simulink model "FF_simulink"  (R2018b)
settings: Solver=VariableStepAuto  StartTime=0.0  StopTime=5  RelTol=1e-3
undefined symbols (not defined in the file): alpha, CL, Cm, g, Iyy, m, V
libraries: vrlib x5, simulink_extras x2
settings Model: Creator=ferra  LastModifiedBy=ferra

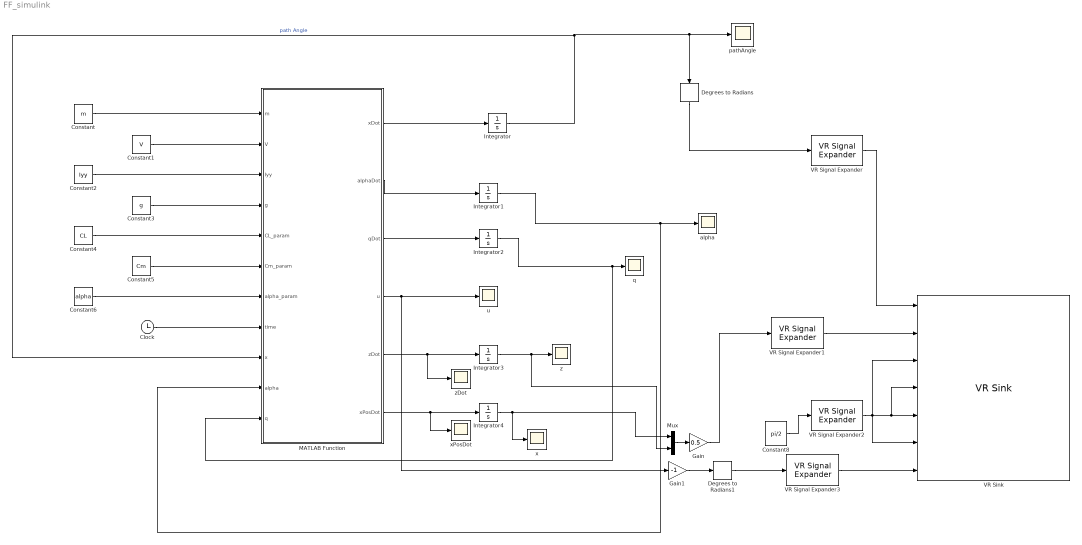
== system FF_simulink ==
  Clock : Clock
  Constant : Constant  Value=m
  Constant1 : Constant  Value=V
  Constant2 : Constant  Value=Iyy
  Constant3 : Constant  Value=g
  Constant4 : Constant  Value=CL
  Constant5 : Constant  Value=Cm
  Constant6 : Constant  Value=alpha
  Constant8 : Constant  Value=pi/2
  Degrees to Radians : simulink_extras/Transformations/Degrees to Radians
  Degrees to Radians1 : simulink_extras/Transformations/Degrees to Radians
  Gain : Gain  Gain=0.5
  Gain1 : Gain  Gain=-1
  Integrator : Integrator
  Integrator1 : Integrator
  Integrator2 : Integrator
  Integrator3 : Integrator  InitialCondition=5
  Integrator4 : Integrator  InitialCondition=-30
  MATLAB Function : MATLAB Function  TreatAsAtomicUnit=on
  Mux : Mux  Inputs=2
  VR Signal Expander : vrlib/VR Signal Expander  outwidth=4  outidx=[4]
      settings: SourceProductName=Simulink 3D Animation  SourceProductBaseCode=VR
  VR Signal Expander1 : vrlib/VR Signal Expander  outwidth=3  outidx=[1 2]
      settings: SourceProductName=Simulink 3D Animation  SourceProductBaseCode=VR
  VR Signal Expander2 : vrlib/VR Signal Expander  outwidth=4  outidx=[4]
      settings: SourceProductName=Simulink 3D Animation  SourceProductBaseCode=VR
  VR Signal Expander3 : vrlib/VR Signal Expander  outwidth=4  outidx=[4]
      settings: SourceProductName=Simulink 3D Animation  SourceProductBaseCode=VR
  VR Sink : vrlib/VR Sink  InstantiateOnLoad=on  SampleTime=0.01  ViewEnable=on  RemoteChange=off  RemoteView=off  FieldsWritten=Airplane.rotation.4.1.1.double#Airplane.translation.3.1.1.double#Rotor_1.rotation.4.1.1.double#Rotor_2.rotation.4.1.1.double#Rotor_3.rotation.4.1.1.double#Rotor_4.rotation.4.1.1.double#Flap_tail.rotation.4.1.1.double  WorldFileName=C:\Users\ferra\Desktop\Projects\Matlab\Thesis\3D-simulation\3D_world.WRL  AutoView=off  VideoDimensions=[]  AllowVariableSize=off
      settings: SourceProductBaseCode=VR
  alpha : Scope
  pathAngle : Scope
  q : Scope
  u : Scope
  x : Scope
  xPosDot : Scope
  "z " : Scope
  zDot : Scope
  wires:
  Constant1/1 -> MATLAB Function/2(V)
  Constant2/1 -> MATLAB Function/3(Iyy)
  Constant3/1 -> MATLAB Function/4(g)
  Constant4/1 -> MATLAB Function/5(CL_param)
  Constant5/1 -> MATLAB Function/6(Cm_param)
  MATLAB Function/1(xDot) -> Integrator/1
  MATLAB Function/2(alphaDot) -> Integrator1/1
  MATLAB Function/3(qDot) -> Integrator2/1
  Integrator/1 -> pathAngle/1, Degrees to Radians/1, MATLAB Function/9(x)  "path Angle"
  Integrator2/1 -> MATLAB Function/11(q), q/1
  Constant6/1 -> MATLAB Function/7(alpha_param)
  MATLAB Function/4(u) -> Gain1/1, u/1
  Clock/1 -> MATLAB Function/8(time)
  Degrees to Radians/1 -> VR Signal Expander/1
  Integrator1/1 -> MATLAB Function/10(alpha), alpha/1
  Constant/1 -> MATLAB Function/1(m)
  MATLAB Function/5(zDot) -> zDot/1, Integrator3/1
  Integrator3/1 -> Mux/2, "z "/1
  MATLAB Function/6(xPosDot) -> xPosDot/1, Integrator4/1
  Integrator4/1 -> Mux/1, x/1
  Mux/1 -> Gain/1
  Gain/1 -> VR Signal Expander1/1
  Constant8/1 -> VR Signal Expander2/1
  VR Signal Expander/1 -> VR Sink/1
  VR Signal Expander1/1 -> VR Sink/2
  VR Signal Expander2/1 -> VR Sink/3, VR Sink/4, VR Sink/5, VR Sink/6
  VR Signal Expander3/1 -> VR Sink/7
  Degrees to Radians1/1 -> VR Signal Expander3/1
  Gain1/1 -> Degrees to Radians1/1

== matlab function FF_simulink/MATLAB Function ==
  data: m input; xDot output; V input; Iyy input; g input; CL_param input; Cm_param input; alpha_param input; time input; alphaDot output; qDot output; x input; alpha input; q input; u output; zDot output; xPosDot output
function [xDot,alphaDot,qDot,u ,zDot , xPosDot ] = FF(m,V,Iyy,g,CL_param,Cm_param,...
                                    alpha_param, time,x,alpha,q)
Cm = mean(Cm_param);
T = 10;


k1 = 2;
k2 = 2;

if(alpha>71)
    alpha = 71;
elseif(alpha<-10)
    alpha = -10;
end



alphaRound = round(alpha*2)/2;

seqIndex = 1:1:length(alpha_param);
index = round(interp1(alpha_param,seqIndex,alphaRound));
CL = CL_param(index);

f = (-g/V) * cos((CL*x)/(m*V));
f1 = (g/V) * cos((CL*x)/(m*V)) - (CL*alpha)/(m*V);
f2 = 0;
g2 = Cm/Iyy;



df_dx =( (g*CL)/(m*V^2) ) * sin((CL*x)/(m*V));
df1_dx = ((-g*CL)/(m*V^2) ) *sin((CL*x)/(m*V));
df_ddx = ((g*CL^2)/(m*V^3)) * cos((CL * x)/(m*V));

%Definition of the xDes
amp = 1;
freq = 2*pi/10;
% xDes = amp * sin(freq*time);

xDes = 15;

e = x-xDes;

% xDesDot = amp *cos(freq*time);
xDesDot = 0;
alphaDes = -f - k1*e + xDesDot; %Virtual : stabilaize the dynamics of x 
alphaDesDot = (-df_dx -k1)*(f+alpha);


e1 = alpha - alphaDes;
qDes = -f1 -x+xDes - k1*e1 + alphaDesDot; %Virtual: stabilize the dynamics of alpha

e2 = q - qDes;

e1Dot = -e - k1*e1 +e2;





d_alphaDesDot_dx = -df_ddx *f - (df_dx)^2 -df_ddx * alpha - k1*df_dx;
par_qDes_x = -df1_dx - 1 + d_alphaDesDot_dx;
par_qDes_e1 = -k1;
qDesDot = par_qDes_x * (f+alpha) + par_qDes_e1 * (e1Dot);
u = (-f2 + qDesDot - e1 - k2*e2)/(g2);

u = sat(u,25);

xDot = f + alpha;
alphaDot = f1 + q;
qDot = f2 + g2 *u;
zDot  = V * sin(deg2rad(x));
xPosDot = V * cos(deg2rad(x));

end
